simulink model "untitled"  (R2025b)
settings: Solver=ode3  StartTime=0.0  StopTime=10  RelTol=1e-3  EnableMultiTasking=on
undefined symbols (not defined in the file): Kv, Kz, Ts
settings Model: FPTRunName=Active  ExtModeTrigDuration=2  Creator=Dell  LastModifiedBy=Dell
settings SolverCC: AlgebraicLoopSolver=TrustRegion
settings DataIOCC: LimitDataPoints=on  SaveFormat=Array
settings OptimizationCC: ReuseModelBlockBuffer=off  ExpressionDepthLimit=2147483647.0  LifeSpan=Inf  MaxStackSize=64
settings DebuggingCC: UnderspecifiedInitializationDetection=Classic  MergeDetectMultiDrivingBlocksExec=none  FcnCallInpInsideContextMsg=warning  UnconnectedInputMsg=warning  UnconnectedOutputMsg=warning  UnconnectedLineMsg=warning  AllowSymbolicDim=off  StateNameClashWarn=warning  SFUnexpectedBacktrackingDiag=warning  SFNoUnconditionalDefaultTransitionDiag=warning  SFExecutionAtInitializationDiag=none  ArithmeticOperatorsInVariantConditions=warning
settings HardwareCC: ProdBitPerInt=16.0  ProdBitPerPointer=16.0  ProdBitPerSizeT=16.0  ProdBitPerPtrDiffT=16.0  ProdLargestAtomicFloat=None  ProdWordSize=8.0  ProdHWDeviceType=Atmel->AVR  UseEmbeddedCoderFeatures=off  UseSimulinkCoderFeatures=off
settings ModelReferenceCC: EnableRefExpFcnMdlSchedulingChecks=on  PropagateSignalLabelsOutOfModel=off
settings SFSimCC: SimUseLocalCustomCode=off  CustomCodeUndefinedFunction=UseInterfaceOnly
settings RTWCC: SystemTargetFile=ert.tlc  HardwareBoard=Arduino Mega 2560  TemplateMakefile=ert_default_tmf  GenerateReport=on  RTWVerbose=off  RTWUseLocalCustomCode=off  Toolchain=Arduino AVR  BuildConfiguration=Faster Runs  LaunchReport=on  GPUComputeCapability=3.5  Description=Embedded Coder
settings CodeAppCC: ForceParamTrailComments=on  OperatorAnnotations=on  StateflowObjectComments=on  MATLABSourceComments=on
settings ERTTargetCC: InlinedParameterPlacement=Hierarchical  DynamicArrayContainerType=coder::array  MultiwordLength=2048.0  ERTCustomFileBanners=off  SupportContinuousTime=on  SupportNonInlinedSFcns=on  RemoveResetFunc=off  ModelStepFunctionPrototypeControlCompliant=off
settings ConfigComp: CovMetricSettings=dw  CovSaveCumulativeToWorkspaceVar=on  CovSaveSingleToWorkspaceVar=on  CovExternalEMLEnable=off  CovSFcnEnable=off

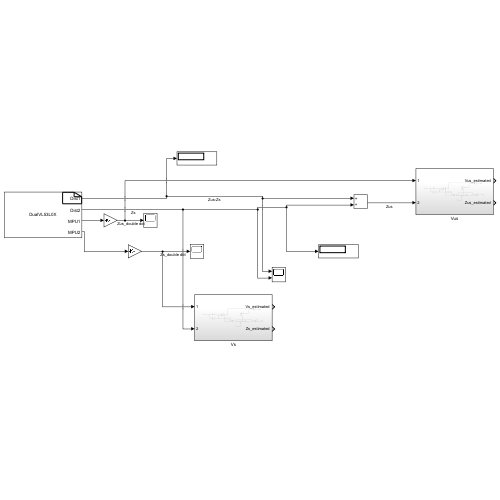
[thumbnail: Simulink's stored preview of the top-level diagram]
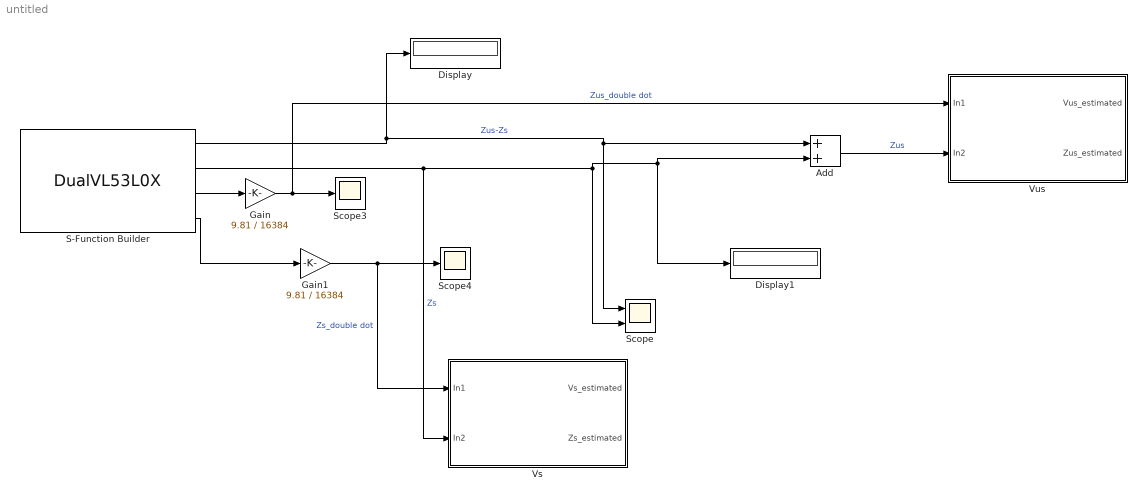
== system untitled ==
  Add : Sum
  Display : Display
  Display1 : Display
  Gain : Gain  Gain=9.81 / 16384
  Gain1 : Gain  Gain=9.81 / 16384
  S-Function Builder : S-Function  FunctionName=DualVL53L0X  SFunctionModules=DualVL53L0X_wrapper.cpp  SFunctionDeploymentMode=off  EnableBusSupport=off  mask(S-Function Builder){}
      mask help: Simulink:masks:SFunctionBuilder_MD
      mask init:
      | val = [[.9  0.75 0.75 1 1 .9 .9 1]',[1 1 0.75 0.75 .9 .9 1 .9]'];try , sys = get_param(gcb,'SfunBuilderFcnName');if isempty(sys), sys = get_param(gcb,'FunctionName'); end,catch, sys = get_param(gcb,'FunctionName'); end
      settings: CopyFcn=set_param(gcbh,'LinkStatus','none')  OpenFcn=sfunctionwizard(gcbh)
      mask Display:
      | plot(val(:,1),val(:,2))
      | disp(sys)
      | port_label('output',1,sprintf('%s', 'Dist1'),'interpreter','tex')
      | port_label('output',2,sprintf('%s', 'Dist2'),'interpreter','tex')
      | port_label('output',3,sprintf('%s', 'MPU1'),'interpreter','tex')
      | port_label('output',4,sprintf('%s', 'MPU2'),'interpreter','tex')
  Scope : Scope  NumInputPorts=2
      settings: ActiveDisplayYMinimum=54.75  ActiveDisplayYMaximum=177.25
  Scope3 : Scope
      settings: ActiveDisplayYMinimum=-5.3696658611297607  ActiveDisplayYMaximum=4.8571286201477051  DataLoggingVariableName=ScopeData3
  Scope4 : Scope
      settings: ActiveDisplayYMinimum=-2.1429565250873566  ActiveDisplayYMaximum=3.0243289768695831  DataLoggingVariableName=ScopeData4
  Vs : Subsystem
  Vus : Subsystem
  wires:
  S-Function Builder/1 -> Display/1, Scope/1, Add/1  "Zus-Zs"
  S-Function Builder/2 -> Vs/2(In2), Add/2, Display1/1, Scope/2  "Zs"
  S-Function Builder/4 -> Gain1/1
  S-Function Builder/3 -> Gain/1
  Gain/1 -> Vus/1(In1), Scope3/1  "Zus_double dot"
  Gain1/1 -> Vs/1(In1), Scope4/1  "Zs_double dot"
  Add/1 -> Vus/2(In2)  "Zus"

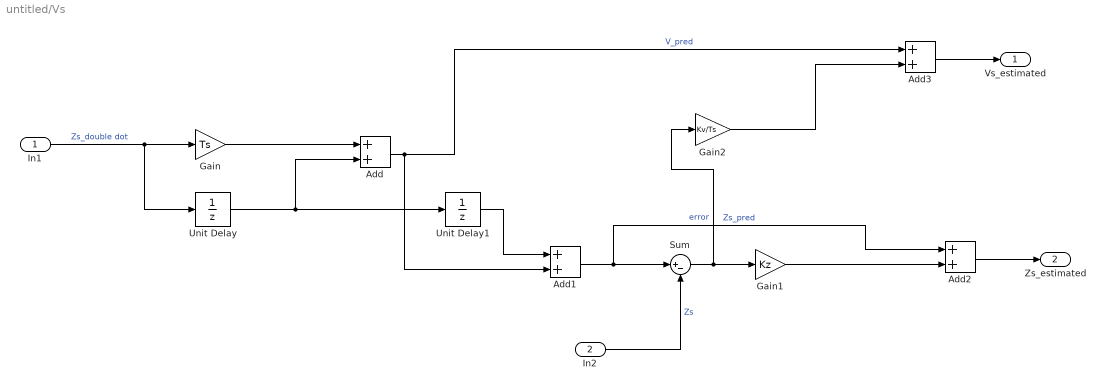
== system untitled/Vs ==
  In1 : Inport
  In2 : Inport  Port=2
  Add{,1..3} (4 alike) : Sum
  Gain : Gain  Gain=Ts
  Gain1 : Gain  Gain=Kz
  Gain2 : Gain  Gain=Kv/Ts
  Sum : Sum  Inputs=|+-
  Unit Delay : UnitDelay  SampleTime=-1  HasFrameUpgradeWarning=on
  Unit Delay1 : UnitDelay  SampleTime=-1  HasFrameUpgradeWarning=on
  "Vs_estimated " : Outport
  "Zs_estimated " : Outport  Port=2
  wires:
  In1/1 -> Unit Delay/1, Gain/1  "Zs_double dot"
  Gain/1 -> Add/1
  Add/1 -> Add3/1, Add1/2  "V_pred"
  Unit Delay/1 -> Unit Delay1/1, Add/2
  Unit Delay1/1 -> Add1/1
  In2/1 -> Sum/2  "Zs"
  Add1/1 -> Add2/1, Sum/1  "Zs_pred"
  Sum/1 -> Gain2/1, Gain1/1  "error"
  Gain1/1 -> Add2/2
  Gain2/1 -> Add3/2
  Add3/1 -> "Vs_estimated "/1
  Add2/1 -> "Zs_estimated "/1

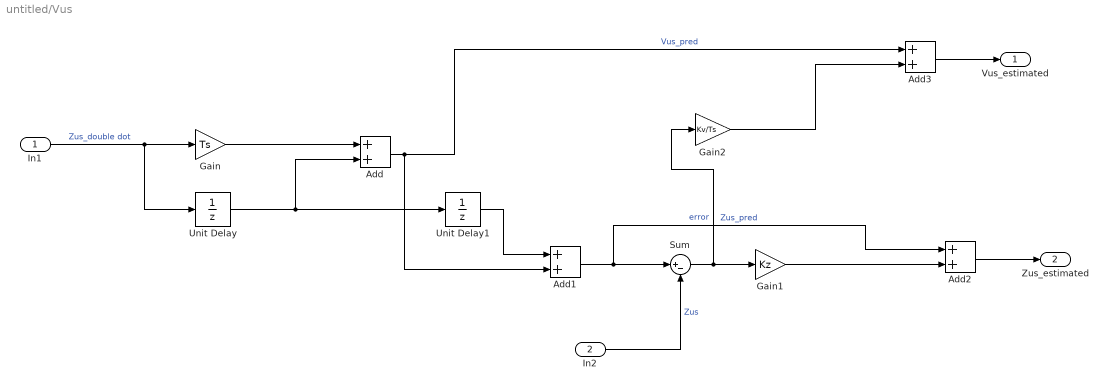
== system untitled/Vus ==
  In1 : Inport
  In2 : Inport  Port=2
  Add{,1..3} (4 alike) : Sum
  Gain : Gain  Gain=Ts
  Gain1 : Gain  Gain=Kz
  Gain2 : Gain  Gain=Kv/Ts
  Sum : Sum  Inputs=|+-
  Unit Delay : UnitDelay  SampleTime=-1  HasFrameUpgradeWarning=on
  Unit Delay1 : UnitDelay  SampleTime=-1  HasFrameUpgradeWarning=on
  "Vus_estimated " : Outport
  "Zus_estimated " : Outport  Port=2
  wires:
  In1/1 -> Unit Delay/1, Gain/1  "Zus_double dot"
  Gain/1 -> Add/1
  Add/1 -> Add3/1, Add1/2  "Vus_pred"
  Unit Delay/1 -> Unit Delay1/1, Add/2
  Unit Delay1/1 -> Add1/1
  In2/1 -> Sum/2  "Zus"
  Add1/1 -> Add2/1, Sum/1  "Zus_pred"
  Sum/1 -> Gain2/1, Gain1/1  "error"
  Gain1/1 -> Add2/2
  Gain2/1 -> Add3/2
  Add3/1 -> "Vus_estimated "/1
  Add2/1 -> "Zus_estimated "/1
